simulink model "simplified"  (R2015b)
settings: Solver=VariableStepAuto  StartTime=0.0  StopTime=100  RelTol=1e-3
libraries: vrlib x2
settings Model: Creator=d_topal  LastModifiedBy=d_topal

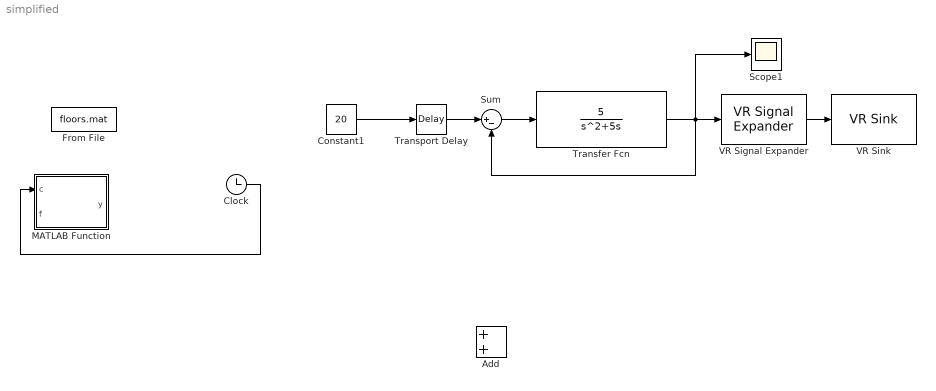
== system simplified ==
  Add : Sum
  Clock : Clock
  Constant1 : Constant  Value=20
  From File : FromFile  FileName=floors.mat  SampleTime=0
  MATLAB Function : MATLAB Function  TreatAsAtomicUnit=on
  Scope1 : Scope
  Sum : Sum  Inputs=|+-
  Transfer Fcn : TransferFcn  Numerator=5  Denominator=[1 5 0]
  Transport Delay : TransportDelay  DelayTime=5
  VR Signal Expander : vrlib/VR Signal Expander  outwidth=3  outidx=[2]
  VR Sink : vrlib/VR Sink  InstantiateOnLoad=on  SampleTime=0.2  ViewEnable=on  RemoteChange=off  RemoteView=off  FieldsWritten=Elevator.translation.3.1.1.double  WorldFileName=world.wrl  AutoView=off  VideoDimensions=[]  AllowVariableSize=off
  wires:
  VR Signal Expander/1 -> VR Sink/1
  Sum/1 -> Transfer Fcn/1
  Transfer Fcn/1 -> VR Signal Expander/1, Scope1/1, Sum/2
  Clock/1 -> MATLAB Function/1(c)
  Transport Delay/1 -> Sum/1
  Constant1/1 -> Transport Delay/1

== matlab function simplified/MATLAB Function ==
  data: y output; c input; f input
function y = fcn(c,f)

for j=2:2:8
    y = j
end

disp(f)
